simulink model "untitled"  (R2022b)
settings: Solver=VariableStepAuto  StartTime=0.0  StopTime=5.0  RelTol=1e-10
undefined symbols (not defined in the file): c, Ig, K, Kn, Kr, l, L, m, OG
libraries: simulink x2
settings Model: Creator=giuliatardito  LastModifiedBy=giuliatardito

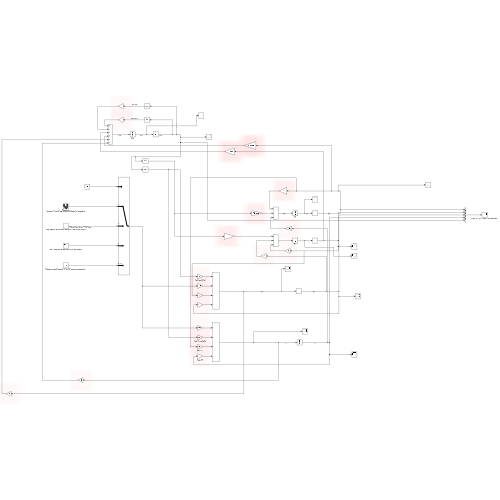
[thumbnail: Simulink's stored preview of the top-level diagram]
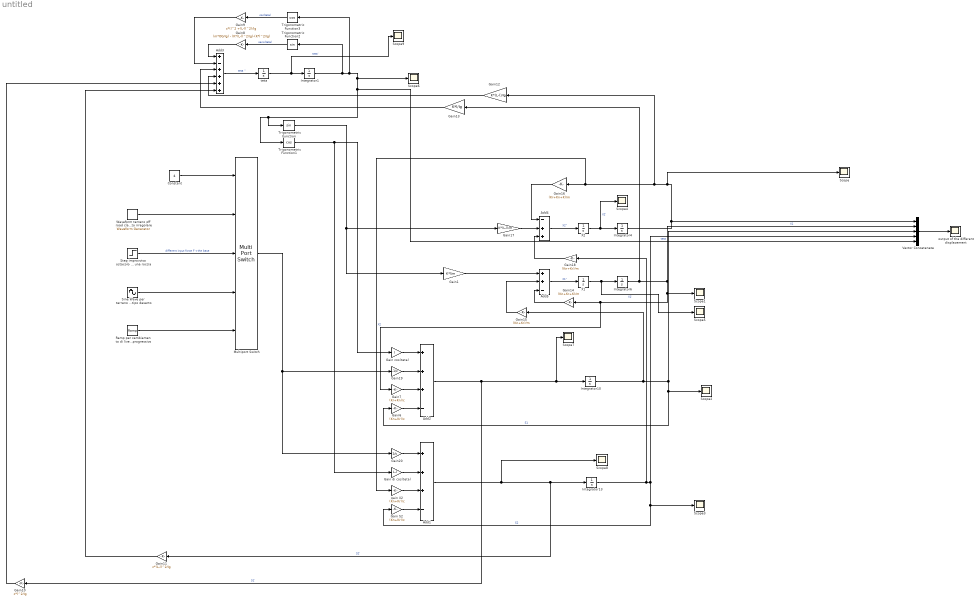
== system untitled ==
  Add1 : Sum  Inputs=+++-
  Add2 : Sum  Inputs=+++-
  Add3 : Sum  Inputs=+-++++
  Add4 : Sum  Inputs=-++
  Add5 : Sum  Inputs=++-
  Constant : Constant  Value=4
  Gain S2 : Gain  Gain=(Kn+Kr)/c
  Gain cos(teta) : Gain  Gain=l
  "Gain di cos(teta) " : Gain  Gain=L-l
  Gain1 : Gain  Gain=K*l/m
  Gain10 : Gain  Gain=c*l^2/Ig
  Gain11 : Gain  Gain=c*(L-l)^2/Ig
  Gain12 : Gain  Gain=K*(L-l)/Ig
  Gain13 : Gain  Gain=K*l/Ig
  Gain14 : Gain  Gain=(Kn+Kr+K)/m
  Gain15 : Gain  Gain=(Kn+Kr)/m
  Gain16 : Gain  Gain=(Kr+Kn+K)/m
  Gain17 : Gain  Gain=K*(L-l)/m
  Gain18 : Gain  Gain=(Kn+Kr)/m
  Gain19 : Gain  Gain=-1/c
  Gain20 : Gain  Gain=1/c
  Gain6 : Gain  Gain=(Kn+Kr)/c
  Gain7 : Gain  Gain=(Kr+Kn)/c
  Gain8 : Gain  Gain=(m*OG/Ig) - (K*(L-l)^2/Ig)-(K*l^2/Ig)
  Gain9 : Gain  Gain=c*(l^2 +(L-l)^2)/Ig
  Integrator{1,4,6,10,13} (5 alike) : Integrator
  Multiport Switch : MultiPortSwitch  Inputs=4  SaturateOnIntegerOverflow=off  InputSameDT=off
  "Ramp per cambiamento di livello terreno progressivo " : simulink/Sources/Ramp  slope=50  start=0  InitialOutput=0
  Scope{,1..9} (10 alike) : Scope
  "Sine Wave per terreno ondulato tipo deserto " : Sin  SampleTime=0
  "Step improvviso ostacolo come un buco o una roccia " : Step  After=500  SampleTime=0
  Trigonometric Function : Trigonometry
  Trigonometric Function1 : Trigonometry  Operator=cos
  Trigonometric Function2 : Trigonometry
  Trigonometric Function3 : Trigonometry  Operator=cos
  Vector Concatenate : Concatenate  NumInputs=5
  "Waveform terreno off road classico con andamento irregolare " : simulink/Sources/Waveform Generator  OutMin=[]  OutMax=[]  OutDataTypeStr=double  RndMeth=Nearest  SelectedSignal=1  Signals=sin(50,100,1)  BlockNames=MultiportSwitch_3dacc86b2160486  SampleTime=0.1
  X1 : Integrator
  X2 : Integrator
  gain X2 : Gain  Gain=(Kn+Kr)/c
  "output of the different displacement " : Scope
  teta : Integrator
  wires:
  teta/1 -> Integrator1/1, Scope9/1  "teta'"
  Integrator1/1 -> Trigonometric Function2/1, Trigonometric Function3/1, Scope6/1, Vector Concatenate/5, Trigonometric Function1/1, Trigonometric Function/1  "teta"
  Trigonometric Function/1 -> Gain1/1, Gain17/1
  Trigonometric Function1/1 -> Gain cos(teta)/1, "Gain di cos(teta) "/1
  X2/1 -> Scope4/1, Integrator4/1  "X2'"
  X1/1 -> Scope5/1, Integrator6/1  "X1'"
  Integrator4/1 -> Scope/1, gain X2/1, Gain16/1, Gain12/1, Vector Concatenate/1  "X2"
  Integrator6/1 -> Gain7/1, Gain14/1, Scope1/1, Vector Concatenate/2, Gain13/1  "X1"
  Add2/1 -> Gain10/1, Scope7/1, Integrator10/1  "S1'"
  Integrator13/1 -> Scope3/1, Gain S2/1, Vector Concatenate/4, Gain18/1  "S2"
  Integrator10/1 -> Gain6/1, Scope2/1, Vector Concatenate/3, Gain15/1  "S1"
  "Gain di cos(teta) "/1 -> Add1/2
  gain X2/1 -> Add1/3
  Gain S2/1 -> Add1/4
  Gain cos(teta)/1 -> Add2/1
  Gain6/1 -> Add2/4
  Gain7/1 -> Add2/3
  Add3/1 -> teta/1  "teta ''"
  Trigonometric Function2/1 -> Gain8/1  "seno(teta)"
  Gain8/1 -> Add3/1
  Trigonometric Function3/1 -> Gain9/1  "cos(teta)"
  Gain9/1 -> Add3/2
  Add1/1 -> Scope8/1, Integrator13/1, Gain11/1  "S2'"
  Gain10/1 -> Add3/5
  Gain11/1 -> Add3/6
  Add4/1 -> X2/1  "X2''"
  Add5/1 -> X1/1  "X1''"
  Gain12/1 -> Add3/4
  Gain13/1 -> Add3/3
  Gain14/1 -> Add5/3
  Gain15/1 -> Add5/2
  Gain16/1 -> Add4/1
  Gain17/1 -> Add4/2
  Gain18/1 -> Add4/3
  Gain19/1 -> Add2/2
  Gain20/1 -> Add1/1
  Vector Concatenate/1 -> "output of the different displacement "/1
  Gain1/1 -> Add5/1
  Constant/1 -> Multiport Switch/1
  "Waveform terreno off road classico con andamento irregolare "/1 -> Multiport Switch/2
  "Step improvviso ostacolo come un buco o una roccia "/1 -> Multiport Switch/3  "different input force F t the base"
  "Sine Wave per terreno ondulato tipo deserto "/1 -> Multiport Switch/4
  "Ramp per cambiamento di livello terreno progressivo "/1 -> Multiport Switch/5
  Multiport Switch/1 -> Gain19/1, Gain20/1
